simulink model "lin_model_PI_MRAC_Sim_CASE2_L1"  (Simulink 7.7)
settings: Solver=ode45  StartTime=0.0  StopTime=TIME  RelTol=1e-3  AbsTol=1e-6
values from neighbouring files (symbols this model uses):
  Am = AA - BB*Kr    [lin_model_LQR.m]    (also in lin_model_PI_MRAC_CASE1.m = Ar-BB*Kr; lin_model_PI_MRAC_CASE1_L1.m = Ar-BB*Kr)
  Ar = Ar_cruise    [parameter.m]
  BB = B_cruise    [parameter.m]
  noise = 0.1    [lin_model_PI_MRAC_CASE1_L1.m]
  omega = 10    [lin_model_PI_MRAC_CASE1_L1.m]
  theta = u(2)    [rigid.m]
  w = randn(size(AA,1),1)    [lin_model_PI_MRAC_CASE1.m]
  x0 = [0;0;0;0]    [beta_crS.m]    (also in flapping.m = []; flappingthrust.m = []; lin_flapping.m = []; lin_model_LQR.m = [3 3 3 0 0 0 0 0 0 0 0]')
  x_hat0 = x0    [lin_model_PI_MRAC_CASE1.m]    (also in lin_model_PI_MRAC_CASE1_L1.m)
undefined symbols (not defined in the file or in its folder): kg, Kr, Ku, PbG
libraries: Projection x3, simulink x2, dspmtrx3 x2
settings Model: Creator=Li  LastModifiedBy=Li  CovHTMLOptions=-aTS=1 -bRG=1 -bTC=1 -hTR=0 -nFC=0 -scm=1 -bcm=1 -xEv=0
settings DataIOCC: LimitDataPoints=off  SaveFormat=StructureWithTime
settings DebuggingCC: SolverPrmCheckMsg=none

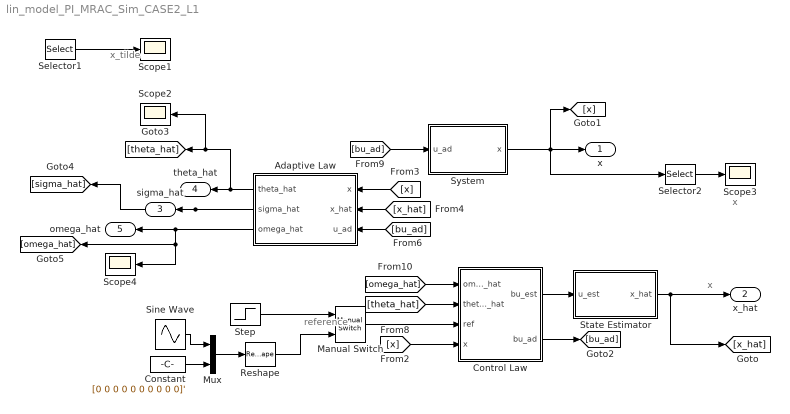
== system lin_model_PI_MRAC_Sim_CASE2_L1 ==
  note: reference
  note: x_tilde
  note: x
  note: x
  Adaptive Law : Subsystem
  Constant : Constant  Value=[0 0 0 0 0 0 0 0 0 0]'
  Control Law : Subsystem
  Manual Switch : simulink/Signal Routing/Manual Switch  SystemSampleTime=-1  sw=1  action=0  varsize=off
  Mux : Mux  Inputs=2
  Reshape : Reshape  OutputDimensionality=Column vector (2-D)
  Scope{1..4} (4 alike) : Scope
      Scope1 settings: TimeRange=3  YMin=-0.4  YMax=2
      Scope2 settings: TimeRange=2  YMin=-0.2  YMax=1.1
      Scope3 settings: TimeRange=2  YMin=-17.5  YMax=12.5  SaveName=ScopeData2
      Scope4 settings: TimeRange=2  YMin=-0.2  YMax=1.1  SaveName=ScopeData3
  Selector1 : Selector  InputPortWidth=11  IndexOptions=Index vector (dialog)  Indices=[1 2 3 4 5]  OutputSizes=1
  Selector2 : Selector  InputPortWidth=11  IndexOptions=Index vector (dialog)  Indices=[1 2 3 4 5]  OutputSizes=1
  Sine Wave : Sin  Amplitude=4  Frequency=2  SampleTime=0
  State Estimator : Subsystem
  Step : Step  Time=0  After=[1 -1 0 0 0 0 0 0 0 0 0]'  SampleTime=0
  System : Subsystem
  x : Outport
  x_hat : Outport  Port=2
  sigma_hat : Outport  Port=3
  theta_hat : Outport  Port=4
  omega_hat : Outport  Port=5
  wires:
  State Estimator/1(x_hat) -> x_hat/1, [x_hat]
  Control Law/1(bu_est) -> State Estimator/1(u_est)
  Control Law/2(bu_ad) -> [bu_ad]
  Step/1 -> Manual Switch/1
  Manual Switch/1 -> Control Law/3(ref)
  Sine Wave/1 -> Mux/1
  Constant/1 -> Mux/2
  Mux/1 -> Reshape/1
  Reshape/1 -> Manual Switch/2
  Selector1/1 -> Scope1/1
  Selector2/1 -> Scope3/1
  [x] -> Control Law/4(x)
  [theta_hat] -> Control Law/2(theta_hat)
  [x] -> Adaptive Law/1(x)
  Adaptive Law/1(theta_hat) -> theta_hat/1, [theta_hat], Scope2/1
  System/1(x) -> x/1, Selector2/1, [x]
  [bu_ad] -> System/1(u_ad)
  [x_hat] -> Adaptive Law/2(x_hat)
  [bu_ad] -> Adaptive Law/3(u_ad)
  Adaptive Law/2(sigma_hat) -> sigma_hat/1, [sigma_hat]
  Adaptive Law/3(omega_hat) -> omega_hat/1, Scope4/1, [omega_hat]
  [omega_hat] -> Control Law/1(omega_hat)

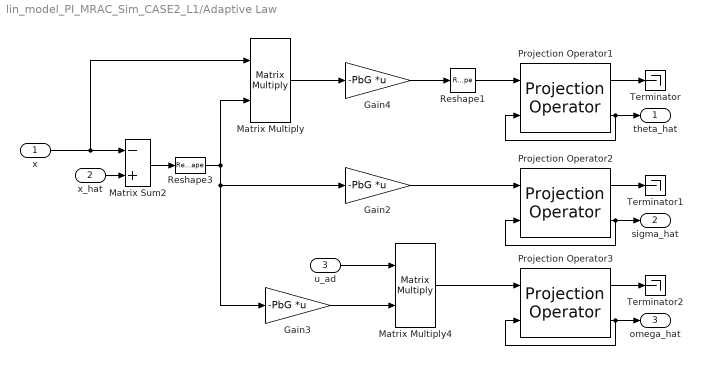
== system lin_model_PI_MRAC_Sim_CASE2_L1/Adaptive Law ==
  x : Inport
  x_hat : Inport  Port=2
  u_ad : Inport  Port=3
  Gain2 : Gain  Gain=-PbG  Multiplication=Matrix(K*u) (u vector)
  Gain3 : Gain  Gain=-PbG  Multiplication=Matrix(K*u) (u vector)
  Gain4 : Gain  Gain=-PbG  Multiplication=Matrix(K*u) (u vector)
  Matrix Sum2 : Sum  Inputs=-+
  Matrix Multiply : Product  Multiplication=Matrix(*)
  Matrix Multiply4 : Product  Multiplication=Matrix(*)
  Projection Operator1 : Projection/Projection Operator  SystemSampleTime=-1  EpsilonTheta=.1  Prmax=bound1  Prcenter=0  Pr0=0
  Projection Operator2 : Projection/Projection Operator  SystemSampleTime=-1  EpsilonTheta=.1  Prmax=bound2  Prcenter=0  Pr0=0
  Projection Operator3 : Projection/Projection Operator  SystemSampleTime=-1  EpsilonTheta=.1  Prmax=bound3  Prcenter=0  Pr0=0
  Reshape1 : Reshape  OutputDimensionality=Column vector (2-D)
  Reshape3 : Reshape  OutputDimensionality=Row vector (2-D)
  Terminator : Terminator
  Terminator1 : Terminator
  Terminator2 : Terminator
  theta_hat : Outport
  sigma_hat : Outport  Port=2
  omega_hat : Outport  Port=3
  wires:
  x/1 -> Matrix Sum2/1, Matrix Multiply/1
  x_hat/1 -> Matrix Sum2/2
  Matrix Sum2/1 -> Reshape3/1
  Reshape3/1 -> Matrix Multiply/2, Gain2/1, Gain3/1
  Matrix Multiply/1 -> Gain4/1
  Gain4/1 -> Reshape1/1
  Reshape1/1 -> Projection Operator1/1
  Projection Operator1/1 -> Terminator/1
  Projection Operator2/1 -> Terminator1/1
  Projection Operator3/1 -> Terminator2/1
  Projection Operator1/2 -> Projection Operator1/2, theta_hat/1
  Gain2/1 -> Projection Operator2/1
  u_ad/1 -> Matrix Multiply4/1
  Gain3/1 -> Matrix Multiply4/2
  Matrix Multiply4/1 -> Projection Operator3/1
  Projection Operator2/2 -> Projection Operator2/2, sigma_hat/1
  Projection Operator3/2 -> Projection Operator3/2, omega_hat/1

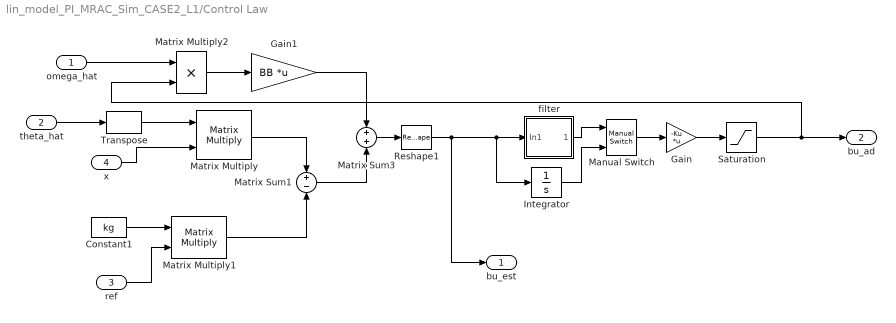
== system lin_model_PI_MRAC_Sim_CASE2_L1/Control Law ==
  omega_hat : Inport
  theta_hat : Inport  Port=2
  ref : Inport  Port=3
  x : Inport  Port=4
  Constant1 : Constant  Value=kg
  Gain : Gain  Gain=-Ku  Multiplication=Matrix(K*u) (u vector)
  Gain1 : Gain  Gain=BB  Multiplication=Matrix(K*u) (u vector)
  Integrator : Integrator  InitialCondition=zeros(11,1)
  Manual Switch : simulink/Signal Routing/Manual Switch  SystemSampleTime=-1  sw=0  action=0  varsize=off
  Matrix Sum1 : Sum  Inputs=+-
  Matrix Sum3 : Sum
  Matrix Multiply : Product  Multiplication=Matrix(*)
  Matrix Multiply1 : Product  Multiplication=Matrix(*)
  Matrix Multiply2 : Product
  Reshape1 : Reshape  OutputDimensionality=Column vector (2-D)
  Saturation : Saturate  UpperLimit=10  LowerLimit=-10
  Transpose : dspmtrx3/Transpose  SystemSampleTime=-1  Hermitian=off  overflowFlag=off
  filter : Subsystem
  bu_est : Outport
  bu_ad : Outport  Port=2
  wires:
  x/1 -> Matrix Multiply/2
  ref/1 -> Matrix Multiply1/2
  Constant1/1 -> Matrix Multiply1/1
  Matrix Multiply/1 -> Matrix Sum1/1
  Matrix Multiply1/1 -> Matrix Sum1/2
  Matrix Sum1/1 -> Matrix Sum3/2
  Gain/1 -> Saturation/1
  Saturation/1 -> bu_ad/1, Matrix Multiply2/2
  Manual Switch/1 -> Gain/1
  filter/1(Out1) -> Manual Switch/1
  Integrator/1 -> Manual Switch/2
  omega_hat/1 -> Matrix Multiply2/1
  theta_hat/1 -> Transpose/1
  Transpose/1 -> Matrix Multiply/1
  Matrix Sum3/1 -> Reshape1/1
  Reshape1/1 -> bu_est/1, filter/1(In1), Integrator/1
  Matrix Multiply2/1 -> Gain1/1
  Gain1/1 -> Matrix Sum3/1

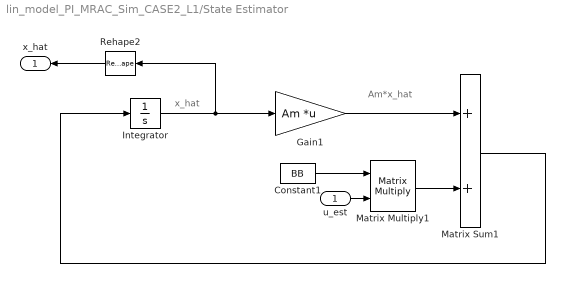
== system lin_model_PI_MRAC_Sim_CASE2_L1/State Estimator ==
  note: x_hat
  note: Am*x_hat
  u_est : Inport
  Constant1 : Constant  Value=BB
  Gain1 : Gain  Gain=Am  Multiplication=Matrix(K*u) (u vector)
  Integrator : Integrator  InitialCondition=x_hat0
  Matrix Sum1 : Sum
  Matrix Multiply1 : Product  Multiplication=Matrix(*)
  Rehape2 : Reshape  OutputDimensionality=Column vector (2-D)
  x_hat : Outport
  wires:
  Integrator/1 -> Gain1/1, Rehape2/1
  Matrix Sum1/1 -> Integrator/1
  Rehape2/1 -> x_hat/1
  u_est/1 -> Matrix Multiply1/2
  Constant1/1 -> Matrix Multiply1/1
  Matrix Multiply1/1 -> Matrix Sum1/2
  Gain1/1 -> Matrix Sum1/1

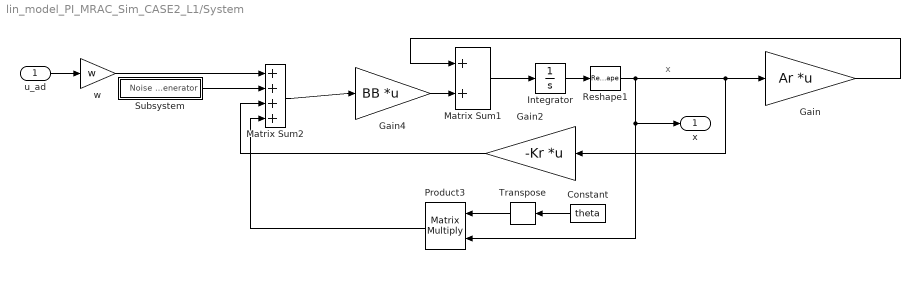
== system lin_model_PI_MRAC_Sim_CASE2_L1/System ==
  note: x
  u_ad : Inport
  Constant : Constant  Value=theta
  Gain : Gain  Gain=Ar  Multiplication=Matrix(K*u) (u vector)
  Gain2 : Gain  Gain=-Kr  Multiplication=Matrix(K*u) (u vector)
  Gain4 : Gain  Gain=BB  Multiplication=Matrix(K*u) (u vector)
  Integrator : Integrator  InitialCondition=x0
  Matrix Sum1 : Sum
  Matrix Sum2 : Sum  Inputs=++++
  Product3 : Product  Multiplication=Matrix(*)  RndMeth=Zero
  Reshape1 : Reshape  OutputDimensionality=Column vector (2-D)
  Subsystem : Subsystem
  Transpose : dspmtrx3/Transpose  SystemSampleTime=-1  Hermitian=off  overflowFlag=off
  w : Gain  Gain=w
  x : Outport
  wires:
  Matrix Sum1/1 -> Integrator/1
  Integrator/1 -> Reshape1/1
  Reshape1/1 -> Gain/1, Gain2/1, x/1, Product3/2
  Gain/1 -> Matrix Sum1/1
  Gain4/1 -> Matrix Sum1/2
  Matrix Sum2/1 -> Gain4/1
  u_ad/1 -> w/1
  w/1 -> Matrix Sum2/1
  Transpose/1 -> Product3/1
  Subsystem/1(Noise Generator) -> Matrix Sum2/2
  Gain2/1 -> Matrix Sum2/3
  Product3/1 -> Matrix Sum2/4
  Constant/1 -> Transpose/1

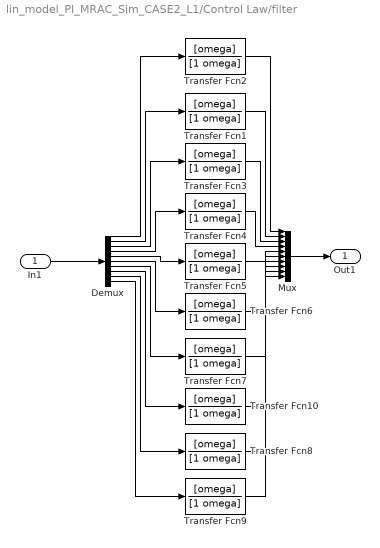
== system lin_model_PI_MRAC_Sim_CASE2_L1/Control Law/filter ==
  In1 : Inport
  Demux : Demux  Outputs=11
  Mux : Mux  Inputs=11
  Transfer Fcn1 : TransferFcn  RequirementInfo={} %GIDa_9d531a5c_f501_426b_9e7c_c695dfc5435a  Numerator=[omega]  Denominator=[1 omega]
  Transfer Fcn10 : TransferFcn  RequirementInfo={} %GIDa_7317762b_9b8c_4ac0_9e52_b61b8e5f0932  Numerator=[omega]  Denominator=[1 omega]
  Transfer Fcn2 : TransferFcn  RequirementInfo={} %GIDa_490594da_e61a_421f_a668_164d100234cb  Numerator=[omega]  Denominator=[1 omega]
  Transfer Fcn3 : TransferFcn  RequirementInfo={} %GIDa_c5ae4f80_59d2_4341_b119_07292f1cab7d  Numerator=[omega]  Denominator=[1 omega]
  Transfer Fcn4 : TransferFcn  RequirementInfo={} %GIDa_626cc1d4_edf9_4907_825d_0a4225b44cdd  Numerator=[omega]  Denominator=[1 omega]
  Transfer Fcn5 : TransferFcn  RequirementInfo={} %GIDa_93886d4a_d3cb_411b_9abc_8ff865cb9b22  Numerator=[omega]  Denominator=[1 omega]
  Transfer Fcn6 : TransferFcn  RequirementInfo={} %GIDa_60575a55_cb95_4a3a_bee5_4fc6950df501  Numerator=[omega]  Denominator=[1 omega]
  Transfer Fcn7 : TransferFcn  RequirementInfo={} %GIDa_57dbe05a_8166_41f7_a8ff_cd8146f79d6f  Numerator=[omega]  Denominator=[1 omega]
  Transfer Fcn8 : TransferFcn  RequirementInfo={} %GIDa_a2616b04_80d9_45b7_8e40_434b57978216  Numerator=[omega]  Denominator=[1 omega]
  Transfer Fcn9 : TransferFcn  RequirementInfo={} %GIDa_bd03ee08_04c1_4911_bc36_58e091c8de11  Numerator=[omega]  Denominator=[1 omega]
  Out1 : Outport
  wires:
  In1/1 -> Demux/1
  Demux/1 -> Transfer Fcn2/1
  Demux/2 -> Transfer Fcn1/1
  Demux/3 -> Transfer Fcn3/1
  Demux/4 -> Transfer Fcn4/1
  Demux/5 -> Transfer Fcn5/1
  Demux/6 -> Transfer Fcn6/1
  Demux/7 -> Transfer Fcn7/1
  Demux/8 -> Transfer Fcn10/1
  Demux/9 -> Transfer Fcn8/1
  Demux/10 -> Transfer Fcn9/1
  Mux/1 -> Out1/1
  Transfer Fcn2/1 -> Mux/1
  Transfer Fcn1/1 -> Mux/2
  Transfer Fcn3/1 -> Mux/3
  Transfer Fcn4/1 -> Mux/4
  Transfer Fcn5/1 -> Mux/5
  Transfer Fcn6/1 -> Mux/6
  Transfer Fcn7/1 -> Mux/7
  Transfer Fcn10/1 -> Mux/8
  Transfer Fcn8/1 -> Mux/9
  Transfer Fcn9/1 -> Mux/10

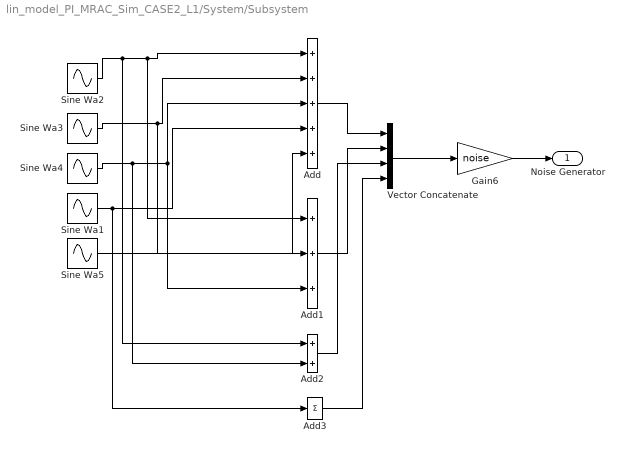
== system lin_model_PI_MRAC_Sim_CASE2_L1/System/Subsystem ==
  Add : Sum  Inputs=+++++
  Add1 : Sum  Inputs=+++
  Add2 : Sum
  Add3 : Sum  Inputs=+
  Gain6 : Gain  Gain=noise
  Sine Wa1 : Sin  Frequency=19  Phase=2  SampleTime=0
  Sine Wa2 : Sin  Frequency=26  Phase=1  SampleTime=0
  Sine Wa3 : Sin  Frequency=23  Phase=0.3  SampleTime=0
  Sine Wa4 : Sin  Frequency=35  Phase=3  SampleTime=0
  Sine Wa5 : Sin  Frequency=25  SampleTime=0
  Vector Concatenate : Concatenate  NumInputs=4  Mode=Vector
  Noise Generator : Outport
  wires:
  Vector Concatenate/1 -> Gain6/1
  Sine Wa2/1 -> Add/1, Add1/1, Add2/1
  Sine Wa3/1 -> Add/2, Add1/2
  Sine Wa4/1 -> Add/3, Add1/3, Add2/2
  Sine Wa1/1 -> Add/4, Add3/1
  Sine Wa5/1 -> Add/5
  Add/1 -> Vector Concatenate/1
  Add1/1 -> Vector Concatenate/2
  Gain6/1 -> Noise Generator/1
  Add2/1 -> Vector Concatenate/3
  Add3/1 -> Vector Concatenate/4
